simulink model "Smart_Grid_2"  (R2024b)
settings: Solver=FixedStepAuto  StartTime=0.0  StopTime=0.5  FixedStep=1e-5  RelTol=1e-3
undefined symbols (not defined in the file): Ion, Lithium
libraries: spsSeriesRLCBranchLib x76, spsRMSLib x65, spsIGBTDiodeLib x41, eeGeneralControl x36, slpidlib x34, spsThreePhaseVIMeasurementLib x32, spsVoltageMeasurementLib x18, simulink x16, spsCurrentMeasurementLib x15, spsThreePhaseBreakerLib x12, spsAlphaBetaZerotodq0Lib x12, spsPower3phPhasorLib x10
(part 2 of 8)

== system Smart_Grid_2/Residential Load 2 ==
  Demux5 : Demux  Outputs=3
  "Power (3ph, Phasor)" : spsPower3phPhasorLib/Power (3ph, Phasor)
      settings: LibrarySourceBlock=|
      | sps_lib/Sensors and Measurements/Power
      | (3ph, Phasor)
  RMS : spsRMSLib/RMS  TrueRMS=on  Freq=60  RMSInit=120  Ts=0
  RMS1 : spsRMSLib/RMS  TrueRMS=on  Freq=60  RMSInit=120  Ts=0
  Relay : Subsystem
  Residential Load 2 : spsThreePhaseParallelRLCLoadLib/Three-Phase Parallel RLC Load  LConnTagsString=A|B|C  Configuration=Y (grounded)  NominalVoltage=25e3  Vabc=[1e3 1e3 1e3]  Vabcp=[1e3 1e3 1e3]  NominalFrequency=50  UnbalancedPower=off  ActivePower=80e3  InductivePower=0  CapacitivePower=5000  Pabc=[10e3 9e3 11e3]  QLabc=[100 90 110]  QCabc=[100 90 110]  Pabcp=[10e3 9e3 11e3]  QLabcp=[100 90 110]  QCabcp=[100 90 110]  Measurements=None  LoadType=constant Z
  Scope : Scope  NumInputPorts=2
  Three-Phase V-I Measurement9 : spsThreePhaseVIMeasurementLib/Three-Phase V-I Measurement  VoltageMeasurement=phase-to-ground  SetLabelV=off  LabelV=Residential_2_Voltage  Vpu=off  VpuLL=off  CurrentMeasurement=yes  SetLabelI=off  LabelI=Residential_2_Current  Ipu=off  Pbase=100e6  Vbase=500e3  OutputType=Complex  PhasorSimulation=off  PSBequivalent=0
  Three-Phase Breaker : spsThreePhaseBreakerLib/Three-Phase Breaker  InitialState=closed  SwitchA=on  SwitchB=on  SwitchC=on  SwitchTimes="[1/60  5/60]"  External=on  BreakerResistance=0.001  SnubberResistance=1e8  SnubberCapacitance=inf  Measurements=Breaker voltages and currents
  Unit Delay2 : UnitDelay  SampleTime=0.001  HasFrameUpgradeWarning=on
  A : PMIOPort  Side=Left
  B : PMIOPort  Port=2  Side=Left
  C : PMIOPort  Port=3  Side=Left
  wires:
  Demux5/1 -> Relay/1(In1)
  Unit Delay2/1 -> Demux5/1
  Three-Phase V-I Measurement9/1 -> "Power (3ph, Phasor)"/1
  Three-Phase V-I Measurement9/2 -> "Power (3ph, Phasor)"/2, Unit Delay2/1
  Demux5/2 -> Relay/2(In2)
  Relay/1(Out1) -> Three-Phase Breaker/1
  "Power (3ph, Phasor)"/2 -> RMS1/1
  Demux5/3 -> Relay/3(In3)
  RMS1/1 -> Scope/2
  "Power (3ph, Phasor)"/1 -> RMS/1
  RMS/1 -> Scope/1
  connections:
  Three-Phase V-I Measurement9/LConn1 -- A/RConn1
  Three-Phase V-I Measurement9/LConn3 -- C/RConn1
  Three-Phase V-I Measurement9/LConn2 -- B/RConn1
  Three-Phase V-I Measurement9/RConn2 -- Three-Phase Breaker/LConn2
  Three-Phase Breaker/RConn2 -- Residential Load 2/LConn2
  Three-Phase Breaker/RConn1 -- Residential Load 2/LConn1
  Three-Phase V-I Measurement9/RConn3 -- Three-Phase Breaker/LConn3
  Three-Phase V-I Measurement9/RConn1 -- Three-Phase Breaker/LConn1
  Three-Phase Breaker/RConn3 -- Residential Load 2/LConn3

== system Smart_Grid_2/Residential Load 3 ==
  Demux5 : Demux  Outputs=3
  "Power (3ph, Phasor)" : spsPower3phPhasorLib/Power (3ph, Phasor)
      settings: LibrarySourceBlock=|
      | sps_lib/Sensors and Measurements/Power
      | (3ph, Phasor)
  RMS : spsRMSLib/RMS  TrueRMS=on  Freq=60  RMSInit=120  Ts=0
  RMS1 : spsRMSLib/RMS  TrueRMS=on  Freq=60  RMSInit=120  Ts=0
  Relay : Subsystem
  Residential Load 3 : spsThreePhaseParallelRLCLoadLib/Three-Phase Parallel RLC Load  LConnTagsString=A|B|C  Configuration=Y (grounded)  NominalVoltage=25e3  Vabc=[1e3 1e3 1e3]  Vabcp=[1e3 1e3 1e3]  NominalFrequency=50  UnbalancedPower=off  ActivePower=50e3  InductivePower=5000  CapacitivePower=0  Pabc=[10e3 9e3 11e3]  QLabc=[100 90 110]  QCabc=[100 90 110]  Pabcp=[10e3 9e3 11e3]  QLabcp=[100 90 110]  QCabcp=[100 90 110]  Measurements=None  LoadType=constant Z
  Scope : Scope  NumInputPorts=2
  Three-Phase V-I Measurement10 : spsThreePhaseVIMeasurementLib/Three-Phase V-I Measurement  VoltageMeasurement=phase-to-ground  SetLabelV=off  LabelV=Residential_3_Voltage  Vpu=off  VpuLL=off  CurrentMeasurement=yes  SetLabelI=off  LabelI=Residential_3_Current  Ipu=off  Pbase=100e6  Vbase=500e3  OutputType=Complex  PhasorSimulation=off  PSBequivalent=0
  Three-Phase Breaker : spsThreePhaseBreakerLib/Three-Phase Breaker  InitialState=closed  SwitchA=on  SwitchB=on  SwitchC=on  SwitchTimes="[1/60  5/60]"  External=on  BreakerResistance=0.001  SnubberResistance=1e8  SnubberCapacitance=inf  Measurements=Breaker voltages and currents
  Unit Delay2 : UnitDelay  SampleTime=0.001  HasFrameUpgradeWarning=on
  A : PMIOPort  Side=Left
  B : PMIOPort  Port=2  Side=Left
  C : PMIOPort  Port=3  Side=Left
  wires:
  Demux5/1 -> Relay/1(In1)
  Unit Delay2/1 -> Demux5/1
  Three-Phase V-I Measurement10/1 -> "Power (3ph, Phasor)"/1
  Three-Phase V-I Measurement10/2 -> "Power (3ph, Phasor)"/2, Unit Delay2/1
  Demux5/2 -> Relay/2(In2)
  Relay/1(Out1) -> Three-Phase Breaker/1
  "Power (3ph, Phasor)"/2 -> RMS1/1
  Demux5/3 -> Relay/3(In3)
  RMS1/1 -> Scope/2
  "Power (3ph, Phasor)"/1 -> RMS/1
  RMS/1 -> Scope/1
  connections:
  Three-Phase V-I Measurement10/LConn3 -- C/RConn1
  Three-Phase V-I Measurement10/LConn2 -- B/RConn1
  Three-Phase V-I Measurement10/LConn1 -- A/RConn1
  Three-Phase Breaker/LConn2 -- Three-Phase V-I Measurement10/RConn2
  Three-Phase Breaker/RConn2 -- Residential Load 3/LConn2
  Three-Phase Breaker/RConn1 -- Residential Load 3/LConn1
  Three-Phase Breaker/LConn3 -- Three-Phase V-I Measurement10/RConn3
  Three-Phase Breaker/LConn1 -- Three-Phase V-I Measurement10/RConn1
  Three-Phase Breaker/RConn3 -- Residential Load 3/LConn3

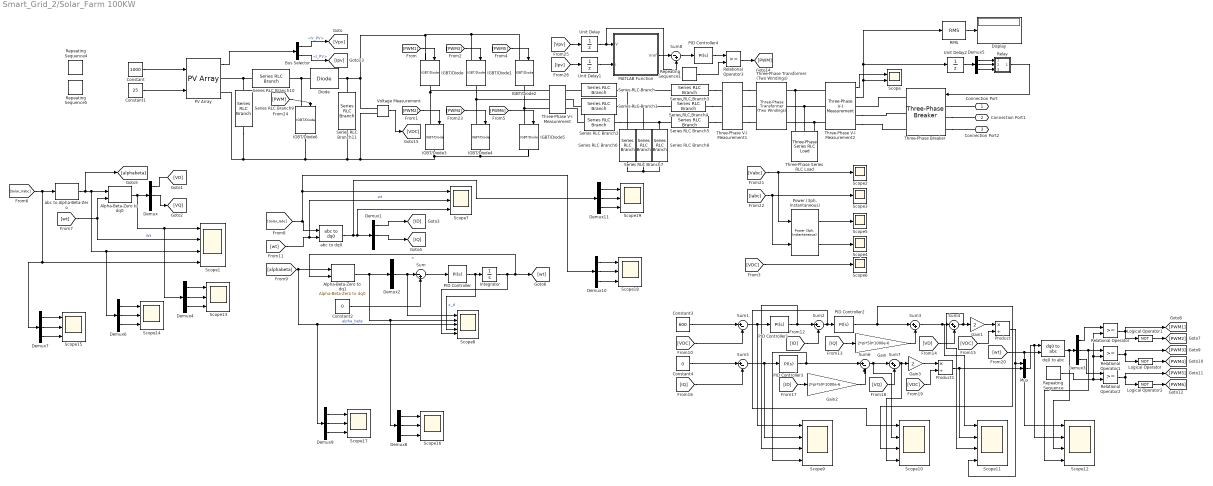
== system Smart_Grid_2/Solar_Farm 100KW ==
  Alpha-Beta-Zero to dq0 : spsAlphaBetaZerotodq0Lib/Alpha-Beta-Zero to dq0  Alignment=90 degrees behind phase A axis
  Alpha-Beta-Zero to dq1 : spsAlphaBetaZerotodq0Lib/Alpha-Beta-Zero to dq0  Alignment=90 degrees behind phase A axis
  Bus Selector : BusSelector  OutputSignals=V_PV,I_PV
  Constant : Constant  Value=1000
  Constant1 : Constant  Value=25
  Constant2 : Constant  Value=0
  Constant3 : Constant  Value=600
  Constant4 : Constant  Value=0
  Demux{,1..11} (12 alike) : Demux  Outputs=3
  Diode : spsDiodeLib/Diode  Ron=0.001  Lon=0  Vf=0.8  IC=0  UseSnubber=0  Rs=500  Cs=250e-9  Measurements=off
  Display : Display
  Gain : Gain  Gain=2*pi*50*1000e-6
  Gain1 : Gain  Gain=2
  Gain2 : Gain  Gain=2*pi*50*1000e-6
  Gain3 : Gain  Gain=2
  IGBT/Diode{,1..6} (7 alike) : spsIGBTDiodeLib/IGBT//Diode  Ron=1e-3  Rs=1e5  Cs=inf  Measurements=off
  Integrator : Integrator
  Logical Operator : Logic  Operator=NOT  AllPortsSameDT=off  OutDataTypeStr=boolean
  Logical Operator1 : Logic  Operator=NOT  AllPortsSameDT=off  OutDataTypeStr=boolean
  Logical Operator2 : Logic  Operator=NOT  AllPortsSameDT=off  OutDataTypeStr=boolean
  MATLAB Function : MATLAB Function  TreatAsAtomicUnit=on
  Mux : Mux  Inputs=3
  PID Controller : slpidlib/PID Controller  Controller=PI  Form=Parallel  TimeDomain=Continuous-time  UseExternalTs=off  SampleTime=-1  IntegratorMethod=Forward Euler  FilterMethod=Forward Euler  ControllerParametersSource=internal  P=10  I=50000  UseKiTs=off  D=0  UseExternalDerivativeSource=off  N=100  UseFilter=on  TunerSelectOption=Transfer Function Based (PID Tuner App)  InitialConditionSource=internal  InitialConditionForIntegrator=0  InitialConditionForFilter=0  DifferentiatorICPrevScaledInput=0  ExternalReset=none  TrackingMode=off  Kt=1  LimitOutput=off  SatLimitsSource=internal  UpperSaturationLimit=inf  LowerSaturationLimit=-inf  LinearizeAsGain=on  AntiWindupMode=none  Kb=1  LimitIntegrator=off  UpperIntegratorSaturationLimit=inf  LowerIntegratorSaturationLimit=-inf  POutMin=[]  POutMax=[]  IOutMin=[]  IOutMax=[]  DOutMin=[]  DOutMax=[]  NOutMin=[]  NOutMax=[]  SumOutMin=[]  SumOutMax=[]  SaturationOutMin=[]  SaturationOutMax=[]  PParamMin=[]  PParamMax=[]  IParamMin=[]  IParamMax=[]  DParamMin=[]  DParamMax=[]  NParamMin=[]  NParamMax=[]  KbParamMin=[]  KbParamMax=[]  KtParamMin=[]  KtParamMax=[]  KbOutMin=[]  KbOutMax=[]  KtOutMin=[]  KtOutMax=[]  IntegratorOutMin=[]  IntegratorOutMax=[]  FilterOutMin=[]  FilterOutMax=[]  SumI1OutMin=[]  SumI1OutMax=[]  SumI2OutMin=[]  SumI2OutMax=[]  SumI3OutMin=[]  SumI3OutMax=[]  SumI4OutMin=[]  SumI4OutMax=[]  SumDOutMin=[]  SumDOutMax=[]  DifferentiatorOutMin=[]  DifferentiatorOutMax=[]  FilterDiffOutCoefMin=[]  FilterDiffOutCoefMax=[]  ReciprocalOutMin=[]  ReciprocalOutMax=[]  SumDenOutMin=[]  SumDenOutMax=[]  SumNumOutMin=[]  SumNumOutMax=[]  DivideOutMin=[]  DivideOutMax=[]  UdiffTsProdOutMin=[]  UdiffTsProdOutMax=[]  NTsProdOutMin=[]  NTsProdOutMax=[]  UintegralTsProdOutMin=[]  UintegralTsProdOutMax=[]  UngainTsProdOutMin=[]  UngainTsProdOutMax=[]  ClampingZeroOutDataTypeStr=Inherit: Inherit via back propagation  ClampingZeroOutMin=[]  ClampingZeroOutMax=[]  FilterDenConstantOutDataTypeStr=Inherit: Inherit via back propagation  FilterDenConstantOutMin=[]  FilterDenConstantOutMax=[]  PCopyOutDataTypeStr=Inherit: Inherit via back propagation  PCopyOutMin=[]  PCopyOutMax=[]  NCopyOutDataTypeStr=Inherit: Inherit via back propagation  NCopyOutMin=[]  NCopyOutMax=[]  IntegratorContinuousStateAttributes=''  IntegratorStateMustResolveToSignalObject=off  IntegratorRTWStateStorageClass=Auto  FilterContinuousStateAttributes=''  FilterStateMustResolveToSignalObject=off  FilterRTWStateStorageClass=Auto  ParallelPVariant=InternalParameters  IdealPVariant=Disabled  IVariant=InternalParameters  DVariant=Disabled  IntegratorVariant=Continuous  SatVariant=Disabled  AWVariant=Passthrough  PCopyVariant=Disabled  TRVariant=Disabled  FdbkBlocksVariant=Forward  IdealPFdbkVariant=Disabled  SatFdbkVariant=Disabled  DerivativeFilterVariant=Disabled  NVariant=Disabled  NCopyVariant=Disabled_SignalSpec  FilterICVariant=Disabled  IntegratorICVariant=InternalICs  ExternalResetVariant=Disabled  TRSumVariant=Passthrough  SumFdbkVariant=Disabled  SumVariant=Sum_PI  TsampFilterVariant=InternalTs  TsampNgainVariant=Passthrough  TsampIntegralVariant=Disabled_SignalSpec  ExternalSaturationOutDataTypeStr=Inherit: Same as second input  DerivativeSourceVariant=Disabled  PreIntVariant=InternalPreInt
  PID Controller1 : slpidlib/PID Controller  Controller=PI  Form=Parallel  TimeDomain=Continuous-time  UseExternalTs=off  SampleTime=-1  IntegratorMethod=Forward Euler  FilterMethod=Forward Euler  ControllerParametersSource=internal  P=0.25  I=300  UseKiTs=off  D=0  UseExternalDerivativeSource=off  N=100  UseFilter=on  TunerSelectOption=Transfer Function Based (PID Tuner App)  InitialConditionSource=internal  InitialConditionForIntegrator=0  InitialConditionForFilter=0  DifferentiatorICPrevScaledInput=0  ExternalReset=none  TrackingMode=off  Kt=1  LimitOutput=off  SatLimitsSource=internal  UpperSaturationLimit=inf  LowerSaturationLimit=-inf  LinearizeAsGain=on  AntiWindupMode=none  Kb=1  LimitIntegrator=off  UpperIntegratorSaturationLimit=inf  LowerIntegratorSaturationLimit=-inf  POutMin=[]  POutMax=[]  IOutMin=[]  IOutMax=[]  DOutMin=[]  DOutMax=[]  NOutMin=[]  NOutMax=[]  SumOutMin=[]  SumOutMax=[]  SaturationOutMin=[]  SaturationOutMax=[]  PParamMin=[]  PParamMax=[]  IParamMin=[]  IParamMax=[]  DParamMin=[]  DParamMax=[]  NParamMin=[]  NParamMax=[]  KbParamMin=[]  KbParamMax=[]  KtParamMin=[]  KtParamMax=[]  KbOutMin=[]  KbOutMax=[]  KtOutMin=[]  KtOutMax=[]  IntegratorOutMin=[]  IntegratorOutMax=[]  FilterOutMin=[]  FilterOutMax=[]  SumI1OutMin=[]  SumI1OutMax=[]  SumI2OutMin=[]  SumI2OutMax=[]  SumI3OutMin=[]  SumI3OutMax=[]  SumI4OutMin=[]  SumI4OutMax=[]  SumDOutMin=[]  SumDOutMax=[]  DifferentiatorOutMin=[]  DifferentiatorOutMax=[]  FilterDiffOutCoefMin=[]  FilterDiffOutCoefMax=[]  ReciprocalOutMin=[]  ReciprocalOutMax=[]  SumDenOutMin=[]  SumDenOutMax=[]  SumNumOutMin=[]  SumNumOutMax=[]  DivideOutMin=[]  DivideOutMax=[]  UdiffTsProdOutMin=[]  UdiffTsProdOutMax=[]  NTsProdOutMin=[]  NTsProdOutMax=[]  UintegralTsProdOutMin=[]  UintegralTsProdOutMax=[]  UngainTsProdOutMin=[]  UngainTsProdOutMax=[]  ClampingZeroOutDataTypeStr=Inherit: Inherit via back propagation  ClampingZeroOutMin=[]  ClampingZeroOutMax=[]  FilterDenConstantOutDataTypeStr=Inherit: Inherit via back propagation  FilterDenConstantOutMin=[]  FilterDenConstantOutMax=[]  PCopyOutDataTypeStr=Inherit: Inherit via back propagation  PCopyOutMin=[]  PCopyOutMax=[]  NCopyOutDataTypeStr=Inherit: Inherit via back propagation  NCopyOutMin=[]  NCopyOutMax=[]  IntegratorContinuousStateAttributes=''  IntegratorStateMustResolveToSignalObject=off  IntegratorRTWStateStorageClass=Auto  FilterContinuousStateAttributes=''  FilterStateMustResolveToSignalObject=off  FilterRTWStateStorageClass=Auto  ParallelPVariant=InternalParameters  IdealPVariant=Disabled  IVariant=InternalParameters  DVariant=Disabled  IntegratorVariant=Continuous  SatVariant=Disabled  AWVariant=Passthrough  PCopyVariant=Disabled  TRVariant=Disabled  FdbkBlocksVariant=Forward  IdealPFdbkVariant=Disabled  SatFdbkVariant=Disabled  DerivativeFilterVariant=Disabled  NVariant=Disabled  NCopyVariant=Disabled_SignalSpec  FilterICVariant=Disabled  IntegratorICVariant=InternalICs  ExternalResetVariant=Disabled  TRSumVariant=Passthrough  SumFdbkVariant=Disabled  SumVariant=Sum_PI  TsampFilterVariant=InternalTs  TsampNgainVariant=Passthrough  TsampIntegralVariant=Disabled_SignalSpec  ExternalSaturationOutDataTypeStr=Inherit: Same as second input  DerivativeSourceVariant=Disabled  PreIntVariant=InternalPreInt
  PID Controller2 : slpidlib/PID Controller  Controller=PI  Form=Parallel  TimeDomain=Continuous-time  UseExternalTs=off  SampleTime=-1  IntegratorMethod=Forward Euler  FilterMethod=Forward Euler  ControllerParametersSource=internal  P=10  I=20  UseKiTs=off  D=0  UseExternalDerivativeSource=off  N=100  UseFilter=on  TunerSelectOption=Transfer Function Based (PID Tuner App)  InitialConditionSource=internal  InitialConditionForIntegrator=0  InitialConditionForFilter=0  DifferentiatorICPrevScaledInput=0  ExternalReset=none  TrackingMode=off  Kt=1  LimitOutput=off  SatLimitsSource=internal  UpperSaturationLimit=inf  LowerSaturationLimit=-inf  LinearizeAsGain=on  AntiWindupMode=none  Kb=1  LimitIntegrator=off  UpperIntegratorSaturationLimit=inf  LowerIntegratorSaturationLimit=-inf  POutMin=[]  POutMax=[]  IOutMin=[]  IOutMax=[]  DOutMin=[]  DOutMax=[]  NOutMin=[]  NOutMax=[]  SumOutMin=[]  SumOutMax=[]  SaturationOutMin=[]  SaturationOutMax=[]  PParamMin=[]  PParamMax=[]  IParamMin=[]  IParamMax=[]  DParamMin=[]  DParamMax=[]  NParamMin=[]  NParamMax=[]  KbParamMin=[]  KbParamMax=[]  KtParamMin=[]  KtParamMax=[]  KbOutMin=[]  KbOutMax=[]  KtOutMin=[]  KtOutMax=[]  IntegratorOutMin=[]  IntegratorOutMax=[]  FilterOutMin=[]  FilterOutMax=[]  SumI1OutMin=[]  SumI1OutMax=[]  SumI2OutMin=[]  SumI2OutMax=[]  SumI3OutMin=[]  SumI3OutMax=[]  SumI4OutMin=[]  SumI4OutMax=[]  SumDOutMin=[]  SumDOutMax=[]  DifferentiatorOutMin=[]  DifferentiatorOutMax=[]  FilterDiffOutCoefMin=[]  FilterDiffOutCoefMax=[]  ReciprocalOutMin=[]  ReciprocalOutMax=[]  SumDenOutMin=[]  SumDenOutMax=[]  SumNumOutMin=[]  SumNumOutMax=[]  DivideOutMin=[]  DivideOutMax=[]  UdiffTsProdOutMin=[]  UdiffTsProdOutMax=[]  NTsProdOutMin=[]  NTsProdOutMax=[]  UintegralTsProdOutMin=[]  UintegralTsProdOutMax=[]  UngainTsProdOutMin=[]  UngainTsProdOutMax=[]  ClampingZeroOutDataTypeStr=Inherit: Inherit via back propagation  ClampingZeroOutMin=[]  ClampingZeroOutMax=[]  FilterDenConstantOutDataTypeStr=Inherit: Inherit via back propagation  FilterDenConstantOutMin=[]  FilterDenConstantOutMax=[]  PCopyOutDataTypeStr=Inherit: Inherit via back propagation  PCopyOutMin=[]  PCopyOutMax=[]  NCopyOutDataTypeStr=Inherit: Inherit via back propagation  NCopyOutMin=[]  NCopyOutMax=[]  IntegratorContinuousStateAttributes=''  IntegratorStateMustResolveToSignalObject=off  IntegratorRTWStateStorageClass=Auto  FilterContinuousStateAttributes=''  FilterStateMustResolveToSignalObject=off  FilterRTWStateStorageClass=Auto  ParallelPVariant=InternalParameters  IdealPVariant=Disabled  IVariant=InternalParameters  DVariant=Disabled  IntegratorVariant=Continuous  SatVariant=Disabled  AWVariant=Passthrough  PCopyVariant=Disabled  TRVariant=Disabled  FdbkBlocksVariant=Forward  IdealPFdbkVariant=Disabled  SatFdbkVariant=Disabled  DerivativeFilterVariant=Disabled  NVariant=Disabled  NCopyVariant=Disabled_SignalSpec  FilterICVariant=Disabled  IntegratorICVariant=InternalICs  ExternalResetVariant=Disabled  TRSumVariant=Passthrough  SumFdbkVariant=Disabled  SumVariant=Sum_PI  TsampFilterVariant=InternalTs  TsampNgainVariant=Passthrough  TsampIntegralVariant=Disabled_SignalSpec  ExternalSaturationOutDataTypeStr=Inherit: Same as second input  DerivativeSourceVariant=Disabled  PreIntVariant=InternalPreInt
  PID Controller3 : slpidlib/PID Controller  Controller=PI  Form=Parallel  TimeDomain=Continuous-time  UseExternalTs=off  SampleTime=-1  IntegratorMethod=Forward Euler  FilterMethod=Forward Euler  ControllerParametersSource=internal  P=10  I=20  UseKiTs=off  D=0  UseExternalDerivativeSource=off  N=100  UseFilter=on  TunerSelectOption=Transfer Function Based (PID Tuner App)  InitialConditionSource=internal  InitialConditionForIntegrator=0  InitialConditionForFilter=0  DifferentiatorICPrevScaledInput=0  ExternalReset=none  TrackingMode=off  Kt=1  LimitOutput=off  SatLimitsSource=internal  UpperSaturationLimit=inf  LowerSaturationLimit=-inf  LinearizeAsGain=on  AntiWindupMode=none  Kb=1  LimitIntegrator=off  UpperIntegratorSaturationLimit=inf  LowerIntegratorSaturationLimit=-inf  POutMin=[]  POutMax=[]  IOutMin=[]  IOutMax=[]  DOutMin=[]  DOutMax=[]  NOutMin=[]  NOutMax=[]  SumOutMin=[]  SumOutMax=[]  SaturationOutMin=[]  SaturationOutMax=[]  PParamMin=[]  PParamMax=[]  IParamMin=[]  IParamMax=[]  DParamMin=[]  DParamMax=[]  NParamMin=[]  NParamMax=[]  KbParamMin=[]  KbParamMax=[]  KtParamMin=[]  KtParamMax=[]  KbOutMin=[]  KbOutMax=[]  KtOutMin=[]  KtOutMax=[]  IntegratorOutMin=[]  IntegratorOutMax=[]  FilterOutMin=[]  FilterOutMax=[]  SumI1OutMin=[]  SumI1OutMax=[]  SumI2OutMin=[]  SumI2OutMax=[]  SumI3OutMin=[]  SumI3OutMax=[]  SumI4OutMin=[]  SumI4OutMax=[]  SumDOutMin=[]  SumDOutMax=[]  DifferentiatorOutMin=[]  DifferentiatorOutMax=[]  FilterDiffOutCoefMin=[]  FilterDiffOutCoefMax=[]  ReciprocalOutMin=[]  ReciprocalOutMax=[]  SumDenOutMin=[]  SumDenOutMax=[]  SumNumOutMin=[]  SumNumOutMax=[]  DivideOutMin=[]  DivideOutMax=[]  UdiffTsProdOutMin=[]  UdiffTsProdOutMax=[]  NTsProdOutMin=[]  NTsProdOutMax=[]  UintegralTsProdOutMin=[]  UintegralTsProdOutMax=[]  UngainTsProdOutMin=[]  UngainTsProdOutMax=[]  ClampingZeroOutDataTypeStr=Inherit: Inherit via back propagation  ClampingZeroOutMin=[]  ClampingZeroOutMax=[]  FilterDenConstantOutDataTypeStr=Inherit: Inherit via back propagation  FilterDenConstantOutMin=[]  FilterDenConstantOutMax=[]  PCopyOutDataTypeStr=Inherit: Inherit via back propagation  PCopyOutMin=[]  PCopyOutMax=[]  NCopyOutDataTypeStr=Inherit: Inherit via back propagation  NCopyOutMin=[]  NCopyOutMax=[]  IntegratorContinuousStateAttributes=''  IntegratorStateMustResolveToSignalObject=off  IntegratorRTWStateStorageClass=Auto  FilterContinuousStateAttributes=''  FilterStateMustResolveToSignalObject=off  FilterRTWStateStorageClass=Auto  ParallelPVariant=InternalParameters  IdealPVariant=Disabled  IVariant=InternalParameters  DVariant=Disabled  IntegratorVariant=Continuous  SatVariant=Disabled  AWVariant=Passthrough  PCopyVariant=Disabled  TRVariant=Disabled  FdbkBlocksVariant=Forward  IdealPFdbkVariant=Disabled  SatFdbkVariant=Disabled  DerivativeFilterVariant=Disabled  NVariant=Disabled  NCopyVariant=Disabled_SignalSpec  FilterICVariant=Disabled  IntegratorICVariant=InternalICs  ExternalResetVariant=Disabled  TRSumVariant=Passthrough  SumFdbkVariant=Disabled  SumVariant=Sum_PI  TsampFilterVariant=InternalTs  TsampNgainVariant=Passthrough  TsampIntegralVariant=Disabled_SignalSpec  ExternalSaturationOutDataTypeStr=Inherit: Same as second input  DerivativeSourceVariant=Disabled  PreIntVariant=InternalPreInt
  PID Controller4 : slpidlib/PID Controller  Controller=PI  Form=Parallel  TimeDomain=Continuous-time  UseExternalTs=off  SampleTime=-1  IntegratorMethod=Forward Euler  FilterMethod=Forward Euler  ControllerParametersSource=internal  P=0.005  I=0.001  UseKiTs=off  D=0  UseExternalDerivativeSource=off  N=100  UseFilter=on  TunerSelectOption=Transfer Function Based (PID Tuner App)  InitialConditionSource=internal  InitialConditionForIntegrator=0  InitialConditionForFilter=0  DifferentiatorICPrevScaledInput=0  ExternalReset=none  TrackingMode=off  Kt=1  LimitOutput=on  SatLimitsSource=internal  UpperSaturationLimit=0.95  LowerSaturationLimit=0  LinearizeAsGain=on  AntiWindupMode=none  Kb=1  LimitIntegrator=off  UpperIntegratorSaturationLimit=inf  LowerIntegratorSaturationLimit=-inf  POutMin=[]  POutMax=[]  IOutMin=[]  IOutMax=[]  DOutMin=[]  DOutMax=[]  NOutMin=[]  NOutMax=[]  SumOutMin=[]  SumOutMax=[]  SaturationOutMin=[]  SaturationOutMax=[]  PParamMin=[]  PParamMax=[]  IParamMin=[]  IParamMax=[]  DParamMin=[]  DParamMax=[]  NParamMin=[]  NParamMax=[]  KbParamMin=[]  KbParamMax=[]  KtParamMin=[]  KtParamMax=[]  KbOutMin=[]  KbOutMax=[]  KtOutMin=[]  KtOutMax=[]  IntegratorOutMin=[]  IntegratorOutMax=[]  FilterOutMin=[]  FilterOutMax=[]  SumI1OutMin=[]  SumI1OutMax=[]  SumI2OutMin=[]  SumI2OutMax=[]  SumI3OutMin=[]  SumI3OutMax=[]  SumI4OutMin=[]  SumI4OutMax=[]  SumDOutMin=[]  SumDOutMax=[]  DifferentiatorOutMin=[]  DifferentiatorOutMax=[]  FilterDiffOutCoefMin=[]  FilterDiffOutCoefMax=[]  ReciprocalOutMin=[]  ReciprocalOutMax=[]  SumDenOutMin=[]  SumDenOutMax=[]  SumNumOutMin=[]  SumNumOutMax=[]  DivideOutMin=[]  DivideOutMax=[]  UdiffTsProdOutMin=[]  UdiffTsProdOutMax=[]  NTsProdOutMin=[]  NTsProdOutMax=[]  UintegralTsProdOutMin=[]  UintegralTsProdOutMax=[]  UngainTsProdOutMin=[]  UngainTsProdOutMax=[]  ClampingZeroOutDataTypeStr=Inherit: Inherit via back propagation  ClampingZeroOutMin=[]  ClampingZeroOutMax=[]  FilterDenConstantOutDataTypeStr=Inherit: Inherit via back propagation  FilterDenConstantOutMin=[]  FilterDenConstantOutMax=[]  PCopyOutDataTypeStr=Inherit: Inherit via back propagation  PCopyOutMin=[]  PCopyOutMax=[]  NCopyOutDataTypeStr=Inherit: Inherit via back propagation  NCopyOutMin=[]  NCopyOutMax=[]  IntegratorContinuousStateAttributes=''  IntegratorStateMustResolveToSignalObject=off  IntegratorRTWStateStorageClass=Auto  FilterContinuousStateAttributes=''  FilterStateMustResolveToSignalObject=off  FilterRTWStateStorageClass=Auto  ParallelPVariant=InternalParameters  IdealPVariant=Disabled  IVariant=InternalParameters  DVariant=Disabled  IntegratorVariant=Continuous  SatVariant=Enabled  AWVariant=Passthrough  PCopyVariant=Disabled  TRVariant=Disabled  FdbkBlocksVariant=Forward  IdealPFdbkVariant=Disabled  SatFdbkVariant=Disabled  DerivativeFilterVariant=Disabled  NVariant=Disabled  NCopyVariant=Disabled_SignalSpec  FilterICVariant=Disabled  IntegratorICVariant=InternalICs  ExternalResetVariant=Disabled  TRSumVariant=Passthrough  SumFdbkVariant=Disabled  SumVariant=Sum_PI  TsampFilterVariant=InternalTs  TsampNgainVariant=Passthrough  TsampIntegralVariant=Disabled_SignalSpec  ExternalSaturationOutDataTypeStr=Inherit: Same as second input  DerivativeSourceVariant=Disabled  PreIntVariant=InternalPreInt
  PV Array : spsPVArrayLib/PV Array  Npar=47  Nser=10  PlotType=array @ 25 deg.C & specified irradiances  S_vec="[ 1000  500  100 ]"  Temp_C_vec="[ 45 25  ]"  ModuleName=Solartech Renewables STR215  PlotWhenSelected=off  Pm=214.963  Ncell=60  Voc=36  Isc=7.73  Vm=28.7  Im=7.49  beta_Voc_pc=-0.41  alpha_Isc_pc=0.05  beta_Voc=-0.1476  alpha_Isc=0.003865  IL=7.8848  I0=1.3153e-09  nI=1.0373  Rsh=5284.6435  Rs=0.36886  RobustModel=off  RobustCellTemperature=313.3991  BAL=on  Tc=1e-6  Tfilter=5e-5
  "Power (3ph, Instantaneous)" : spsPower3phInstantaneousLib/Power (3ph, Instantaneous)
  Product : Product  Inputs=*/
  Product1 : Product  Inputs=*/
  RMS : spsRMSLib/RMS  TrueRMS=on  Freq=50  RMSInit=0  Ts=0.001
  Relational Operator{,1..3} (4 alike) : RelationalOperator  OutDataTypeStr=boolean  RndMeth=Simplest  InputSameDT=off
  Relay : Subsystem
  Repeating Sequence : simulink/Sources/Repeating Sequence  rep_seq_t=[0 0.00005 0.0001]  rep_seq_y=[-1 1 -1]
  Repeating Sequence1 : simulink/Sources/Repeating Sequence  rep_seq_t=[0 0.0002]  rep_seq_y=[0 1]
  Repeating Sequence4 : simulink/Sources/Repeating Sequence  rep_seq_t=|  rep_seq_y=|
      rep_seq_t=|
      | [0
      | 0.050505051
      | 0.101010101
      | 0.151515152
      | 0.202020202
      | 0.252525253
      | 0.303030303
      | 0.353535354
      | 0.404040404
      | 0.454545455
      | 0.505050505
      | 0.555555556
      | 0.606060606
      | 0.656565657
      | 0.707070707
      | 0.757575758
      | 0.808080808
      | 0.858585859
      | 0.909090909
      | 0.95959596
      | 1.01010101
      | 1.060606061
      | 1.111111111
      | 1.161616162
      | 1.212121212
      | 1.262626263
      | 1.313131313
      | 1.363636364
      | 1.414141414
      | 1.464646465
      | 1.515151515
      | 1.565656566
      | 1.616161616
      | 1.666666667
      | 1.717171717
      | 1.767676768
      | 1.818181818
      | 1.868686869
      | 1.919191919
      | 1.96969697
      | 2.02020202
      | 2.070707071
      | 2.121212121
      | 2.171717172
      | 2.222222222
      | 2.272727273
      | 2.323232323
      | 2.373737374
      | 2.424242424
      | 2.474747475
      | 2.525252525
      | 2.575757576
      | 2.626262626
      | 2.676767677
      | 2.727272727
      | 2.777777778
      | 2.828282828
      | 2.878787879
      | 2.929292929
      | 2.97979798
      | 3.03030303
      | 3.080808081
      | 3.131313131
      | 3.181818182
      | 3.232323232
      | 3.282828283
      | 3.333333333
      | 3.383838384
      | 3.434343434
      | 3.484848485
      | 3.535353535
      | 3.585858586
      | 3.636363636
      | 3.686868687
      | 3.737373737
      | 3.787878788
      | 3.838383838
      | 3.888888889
      | 3.939393939
      | 3.98989899
      | 4.04040404
      | 4.090909091
      | 4.141414141
      | 4.191919192
      | 4.242424242
      | 4.292929293
      | 4.343434343
      | 4.393939394
      | 4.444444444
      | 4.494949495
      | 4.545454545
      | 4.595959596
      | 4.646464646
      | 4.696969697
      | 4.747474747
      | 4.797979798
      | 4.848484848
      | 4.898989899
      | 4.949494949
      | 5
      | ]
      rep_seq_y=|
      | [961.731225
      | 1045.11045
      | 1008.510311
      | 931.1104746
      | 1078.747978
      | 1059.848715
      | 904.7074666
      | 958.4820041
      | 947.434516
      | 1200.30114
      | 1066.976539
      | 1076.06026
      | 1093.154951
      | 1055.443451
      | 901.2390038
      | 1091.945745
      | 953.8403505
      | 0
      | 0
      | 0
      | 0
      | 0
      | 0
      | 0
      | 1000.207161
      | 1038.593515
      | 941.0686417
      | 500.4919759
      | 550.6758168
      | 939.0750316
      | 936.755036
      | 1086.548091
      | 1027.661514
      | 1076.95396
      | 1093.908545
      | 969.8802795
      | 900.0079837
      | 1039.498473
      | 350.3719924
      | 400.3916341
      | 420.2982665
      | 1029.138637
      | 960.2858986
      | 949.2673312
      | 1067.379392
      | 1058.456925
      | 986.3566657
      | 948.4318496
      | 942.3822613
      | 916.4479292
      | 1002.255686
      | 1068.546297
      | 1080.245726
      | 927.5500873
      | 967.3817546
      | 946.7661715
      | 998.0233465
      | 1036.639395
      | 1075.77624
      | 1099.604998
      | 910.8779584
      | 1053.351328
      | 1079.393791
      | 1002.654666
      | 1028.287667
      | 951.1786685
      | 974.5537092
      | 1024.300777
      | 998.6087208
      | 903.7161662
      | 1081.108921
      | 922.113608
      | 923.529757
      | 941.6210422
      | 984.1534846
      | 1046.704566
      | 1087.490012
      | 917.4050569
      | 1068.395551
      | 984.3349603
      | 1054.093286
      | 999.8107273
      | 917.4038553
      | 932.1890541
      | 951.4940944
      | 903.1694839
      | 964.5157871
      | 917.1253389
      | 954.3180431
      | 1071.497523
      | 935.2374128
      | 1056.905007
      | 1039.774892
      | 1055.449509
      | 984.8677414
      | 961.3374658
      | 1088.467992
      | 1058.226697
      | 970.9178907
      | 908.7847737
      | ]
  Repeating Sequence5 : simulink/Sources/Repeating Sequence  rep_seq_t=|  rep_seq_y=|
      rep_seq_t=|
      | [0
      | 0.050505051
      | 0.101010101
      | 0.151515152
      | 0.202020202
      | 0.252525253
      | 0.303030303
      | 0.353535354
      | 0.404040404
      | 0.454545455
      | 0.505050505
      | 0.555555556
      | 0.606060606
      | 0.656565657
      | 0.707070707
      | 0.757575758
      | 0.808080808
      | 0.858585859
      | 0.909090909
      | 0.95959596
      | 1.01010101
      | 1.060606061
      | 1.111111111
      | 1.161616162
      | 1.212121212
      | 1.262626263
      | 1.313131313
      | 1.363636364
      | 1.414141414
      | 1.464646465
      | 1.515151515
      | 1.565656566
      | 1.616161616
      | 1.666666667
      | 1.717171717
      | 1.767676768
      | 1.818181818
      | 1.868686869
      | 1.919191919
      | 1.96969697
      | 2.02020202
      | 2.070707071
      | 2.121212121
      | 2.171717172
      | 2.222222222
      | 2.272727273
      | 2.323232323
      | 2.373737374
      | 2.424242424
      | 2.474747475
      | 2.525252525
      | 2.575757576
      | 2.626262626
      | 2.676767677
      | 2.727272727
      | 2.777777778
      | 2.828282828
      | 2.878787879
      | 2.929292929
      | 2.97979798
      | 3.03030303
      | 3.080808081
      | 3.131313131
      | 3.181818182
      | 3.232323232
      | 3.282828283
      | 3.333333333
      | 3.383838384
      | 3.434343434
      | 3.484848485
      | 3.535353535
      | 3.585858586
      | 3.636363636
      | 3.686868687
      | 3.737373737
      | 3.787878788
      | 3.838383838
      | 3.888888889
      | 3.939393939
      | 3.98989899
      | 4.04040404
      | 4.090909091
      | 4.141414141
      | 4.191919192
      | 4.242424242
      | 4.292929293
      | 4.343434343
      | 4.393939394
      | 4.444444444
      | 4.494949495
      | 4.545454545
      | 4.595959596
      | 4.646464646
      | 4.696969697
      | 4.747474747
      | 4.797979798
      | 4.848484848
      | 4.898989899
      | 4.949494949
      | 5
      | ]
      rep_seq_y=|
      | [39.09040776
      | 33.78587594
      | 22.64735033
      | 39.07287359
      | 39.6979768
      | 38.77147184
      | 20.1126813
      | 32.72378376
      | 39.96246483
      | 35.82177272
      | 20.49274147
      | 30.62419618
      | 26.17597826
      | 38.66721226
      | 21.62717688
      | 21.97818325
      | 38.49825769
      | 36.17310767
      | 26.07943066
      | 28.57378964
      | 21.24308492
      | 26.36590257
      | 30.33391133
      | 29.99686413
      | 23.22998026
      | 38.53716796
      | 34.59986631
      | 24.14165098
      | 22.46973707
      | 25.64228662
      | 26.2700476
      | 38.78343151
      | 22.35947723
      | 26.17383265
      | 34.52437963
      | 27.85768308
      | 24.96183533
      | 24.06305535
      | 34.13520509
      | 29.27960727
      | 34.02958238
      | 31.19691976
      | 29.65246289
      | 22.82071168
      | 26.36562902
      | 37.00153111
      | 35.65458064
      | 23.04842989
      | 21.32587473
      | 30.35583122
      | 25.41212742
      | 32.94902261
      | 31.40546329
      | 27.39813642
      | 25.32840072
      | 24.51675606
      | 24.01324349
      | 30.88693234
      | 29.85790683
      | 27.80551597
      | 23.11303618
      | 30.90103153
      | 38.1204096
      | 37.66129424
      | 32.54190455
      | 25.87105192
      | 30.81157353
      | 33.91804655
      | 31.05518166
      | 37.05481269
      | 24.91683857
      | 28.99411247
      | 30.36584588
      | 22.30935985
      | 25.91476526
      | 21.87306052
      | 36.26770138
      | 23.15482256
      | 32.66810495
      | 33.93954581
      | 32.63846158
      | 28.38171681
      | 23.17522821
      | 25.70852908
      | 32.50154208
      | 34.83572597
      | 33.50995143
      | 36.59220243
      | 39.49654504
      | 26.69276484
      | 30.47625268
      | 24.22660242
      | 28.84239867
      | 24.12405795
      | 22.94119138
      | 22.51756848
      | 29.72937034
      | 31.48890937
      | 25.32014349
      | 20.45980854
      | ]
  Scope : Scope  NumInputPorts=2
  Scope{1,9..12} (5 alike) : Scope  NumInputPorts=4
  Scope{7,13..19} (8 alike) : Scope  NumInputPorts=3
  Scope{2..6} (5 alike) : Scope
  Scope8 : Scope  NumInputPorts=5
  Series RLC Branch{,1..5} (6 alike) : spsSeriesRLCBranchLib/Series RLC Branch  LConnTagsString=__new0  RConnTagsString=__new0  BranchType=RL  Resistance=1e-3  Inductance=500e-6  SetiL0=off  InitialCurrent=0  Capacitance=1e-6  Setx0=off  InitialVoltage=0  Measurements=None
  Series RLC Branch10 : spsSeriesRLCBranchLib/Series RLC Branch  LConnTagsString=__new0  RConnTagsString=__new0  BranchType=L  Resistance=1e-3  Inductance=1.45e-3  SetiL0=off  InitialCurrent=0  Capacitance=1000e-6  Setx0=off  InitialVoltage=0  Measurements=None
  Series RLC Branch11 : spsSeriesRLCBranchLib/Series RLC Branch  LConnTagsString=__new0  RConnTagsString=__new0  BranchType=C  Resistance=1e-3  Inductance=3227e-3  SetiL0=off  InitialCurrent=0  Capacitance=3227e-6  Setx0=off  InitialVoltage=0  Measurements=None
  Series RLC Branch6 : spsSeriesRLCBranchLib/Series RLC Branch  LConnTagsString=__new0  RConnTagsString=__new0  BranchType=RC  Resistance=1e-3  Inductance=500e-6  SetiL0=off  InitialCurrent=0  Capacitance=100e-6  Setx0=off  InitialVoltage=0  Measurements=None
  Series RLC Branch7 : spsSeriesRLCBranchLib/Series RLC Branch  LConnTagsString=__new0  RConnTagsString=__new0  BranchType=RC  Resistance=1e-3  Inductance=500e-6  SetiL0=off  InitialCurrent=0  Capacitance=100e-6  Setx0=off  InitialVoltage=0  Measurements=None
  Series RLC Branch8 : spsSeriesRLCBranchLib/Series RLC Branch  LConnTagsString=__new0  RConnTagsString=__new0  BranchType=RC  Resistance=1e-3  Inductance=500e-6  SetiL0=off  InitialCurrent=0  Capacitance=100e-6  Setx0=off  InitialVoltage=0  Measurements=None
  Series RLC Branch9 : spsSeriesRLCBranchLib/Series RLC Branch  LConnTagsString=__new0  RConnTagsString=__new0  BranchType=RC  Resistance=1e-3  Inductance=1e-3  SetiL0=off  InitialCurrent=0  Capacitance=100e-6  Setx0=off  InitialVoltage=0  Measurements=None
  Sum : Sum  Inputs=|-+
  Sum{1..2,5..6} (4 alike) : Sum  Inputs=|+-
  Sum3 : Sum  Inputs=|++
  Sum4 : Sum  Inputs=|++
  Sum7 : Sum  Inputs=|++
  Sum8 : Sum  Inputs=|-+
  Three-Phase Series RLC Load : spsThreePhaseSeriesRLCLoadLib/Three-Phase Series RLC Load  LConnTagsString=A|B|C  Configuration=Y (grounded)  NominalVoltage=25e3  Vabc=[1e3 1e3 1e3]  Vabcp=[1e3 1e3 1e3]  NominalFrequency=50  UnbalancedPower=off  ActivePower=100  InductivePower=0  CapacitivePower=10000  Pabc=[10e3 9e3 11e3]  QLabc=[100 90 110]  QCabc=[100 90 110]  Pabcp=[10e3 9e3 11e3]  QLabcp=[100 90 110]  QCabcp=[100 90 110]  Measurements=None  LoadType=constant Z
  Three-Phase Transformer (Two Windings) : spsThreePhaseTransformerTwoWindingsLib/Three-Phase Transformer (Two Windings)  Winding1Connection=Yg  Winding2Connection=Yg  CoreType=Three single-phase transformers  SetSaturation=off  Hysteresis=off  DataFile='hysteresis'  SetInitialFlux=off  Measurements=None  UNITS=pu  NominalPower=[ 25e6 , 50 ]  Winding1=[ 400 , 0 , 0 ]  Winding2=[ 25e3 , 0 , 0 ]  Rm=500  Lm=500  L0=0.5  Saturation=[ 0,0 ; 0.0024,1.2 ; 1.0,1.52 ]  InitialFluxes=[ 0.8 , -0.8 , 0.7 ]  BreakLoop=off  DiscreteSolver=Trapezoidal iterative  DataType=off  TransfoNumber=1
  Three-Phase V-I Measurement : spsThreePhaseVIMeasurementLib/Three-Phase V-I Measurement  VoltageMeasurement=no  SetLabelV=off  LabelV=Vabc  Vpu=off  VpuLL=off  CurrentMeasurement=yes  SetLabelI=on  LabelI=Solar_Iabc  Ipu=off  Pbase=100e6  Vbase=500e3  OutputType=Complex  PhasorSimulation=off  PSBequivalent=0
  Three-Phase V-I Measurement1 : spsThreePhaseVIMeasurementLib/Three-Phase V-I Measurement  VoltageMeasurement=phase-to-ground  SetLabelV=on  LabelV=Solar_Vabc  Vpu=off  VpuLL=off  CurrentMeasurement=no  SetLabelI=off  LabelI=Iabc  Ipu=off  Pbase=100e6  Vbase=500e3  OutputType=Complex  PhasorSimulation=off  PSBequivalent=0
  Three-Phase V-I Measurement2 : spsThreePhaseVIMeasurementLib/Three-Phase V-I Measurement  VoltageMeasurement=phase-to-ground  SetLabelV=off  LabelV=Vabc  Vpu=off  VpuLL=off  CurrentMeasurement=yes  SetLabelI=off  LabelI=Iabc  Ipu=off  Pbase=100e6  Vbase=500e3  OutputType=Complex  PhasorSimulation=off  PSBequivalent=0
  Three-Phase Breaker : spsThreePhaseBreakerLib/Three-Phase Breaker  InitialState=closed  SwitchA=on  SwitchB=on  SwitchC=on  SwitchTimes="[1/60  5/60]"  External=on  BreakerResistance=0.001  SnubberResistance=1e8  SnubberCapacitance=inf  Measurements=Breaker voltages and currents
  Unit Delay : UnitDelay  SampleTime=1e-4  HasFrameUpgradeWarning=on
  Unit Delay1 : UnitDelay  SampleTime=1e-4  HasFrameUpgradeWarning=on
  Unit Delay2 : UnitDelay  SampleTime=0.001  HasFrameUpgradeWarning=on
  Voltage Measurement : spsVoltageMeasurementLib/Voltage Measurement  PhasorSimulation=off  OutputType=Complex  PSBequivalent=0
  abc to Alpha-Beta-Zero : spsabctoAlphaBetaZeroLib/abc to Alpha-Beta-Zero
  abc to dq0 : spsabctodq0Lib/abc to dq0  Alignment=90 degrees behind phase A axis
  dq0 to abc : spsdq0toabcLib/dq0 to abc  Alignment=90 degrees behind phase A axis
  Connection Port : PMIOPort  Side=Right
  Connection Port1 : PMIOPort  Port=2  Side=Right
  Connection Port2 : PMIOPort  Port=3  Side=Right
  wires:
  Three-Phase V-I Measurement2/1 -> Scope/1
  [VDC] -> Scope6/1
  [Vabc] -> Scope2/1, "Power (3ph, Instantaneous)"/1
  "Power (3ph, Instantaneous)"/1 -> Scope5/1
  "Power (3ph, Instantaneous)"/2 -> Scope4/1
  [Iabc] -> Scope3/1, "Power (3ph, Instantaneous)"/2
  Demux3/3 -> Relational Operator2/1
  Repeating Sequence/1 -> Relational Operator/2, Relational Operator1/2, Relational Operator2/2
  Demux3/1 -> Relational Operator/1
  Demux3/2 -> Scope12/4, Relational Operator1/1
  dq0 to abc/1 -> Scope12/3, Demux3/1
  [ID] -> Gain2/1
  [VDC] -> Product1/2
  Sum5/1 -> Scope9/2, PID Controller3/1
  Constant4/1 -> Sum5/1
  [IQ] -> Sum5/2
  Sum6/1 -> Scope10/2, Sum7/1
  Sum7/1 -> Scope10/4, Gain3/1
  PID Controller3/1 -> Scope9/4, Sum6/1
  [VQ] -> Sum7/2
  Gain2/1 -> Sum6/2
  Gain3/1 -> Product1/1
  Demux2/2 -> Scope8/1, Sum/1
  [alphabeta] -> Demux9/1, Scope8/3, Alpha-Beta-Zero to dq1/1  "alpha_beta"
  Integrator/1 -> Scope8/5, Alpha-Beta-Zero to dq1/2, [wt]  "x"
  Constant2/1 -> Sum/2
  Sum/1 -> PID Controller/1
  PID Controller/1 -> Scope8/4, Integrator/1  "x_d"
  Demux1/2 -> [IQ]
  [Solar_Iabc] -> Demux10/1, Scope7/1, abc to dq0/1
  [wt] -> Scope7/2, abc to dq0/2  "wt"
  Demux1/1 -> [ID]
  PID Controller1/1 -> Scope9/3, Sum2/1
  Sum2/1 -> Scope10/1, PID Controller2/1
  [VDC] -> Sum1/2
  [VD] -> Sum4/2
  PID Controller2/1 -> Scope10/3, Sum3/1
  Sum3/1 -> Scope11/1, Sum4/1
  [IQ] -> Gain/1
  [VDC] -> Product/2
  Constant3/1 -> Sum1/1
  Gain/1 -> Sum3/2
  [ID] -> Sum2/2
  Gain1/1 -> Product/1
  Sum4/1 -> Scope11/3, Gain1/1
  Sum1/1 -> Scope9/1, PID Controller1/1
  Demux/1 -> [VD]
  Alpha-Beta-Zero to dq0/1 -> Demux/1, Demux4/1, Scope1/1
  [wt] -> Scope1/2, Alpha-Beta-Zero to dq0/2  "Wt"
  Demux/2 -> [VQ]
  Product1/1 -> Scope11/2, Mux/2
  Product/1 -> Scope11/4, Mux/1
  Mux/1 -> Scope12/2, dq0 to abc/1
  [wt] -> Scope12/1, dq0 to abc/2
  Logical Operator1/1 -> [PWM2]
  Logical Operator2/1 -> [PWM6]
  Relational Operator2/1 -> Logical Operator2/1, [PWM5]
  Relational Operator/1 -> Logical Operator1/1, [PWM1]
  Logical Operator/1 -> [PWM4]
  Relational Operator1/1 -> [PWM3], Logical Operator/1
  [PWM1] -> IGBT/Diode/1
  [PWM5] -> IGBT/Diode2/1
  [PWM4] -> IGBT/Diode4/1
  [PWM3] -> IGBT/Diode1/1
  [PWM6] -> IGBT/Diode5/1
  [PWM2] -> IGBT/Diode3/1
  Voltage Measurement/1 -> [VDC]
  Relational Operator3/1 -> [PWM]
  Sum8/1 -> PID Controller4/1
  [Ipv] -> Unit Delay1/1
  Repeating Sequence1/1 -> Relational Operator3/2
  Unit Delay/1 -> Sum8/2, MATLAB Function/1(V)
  [PWM] -> IGBT/Diode6/1
  PID Controller4/1 -> Relational Operator3/1
  PV Array/1 -> Bus Selector/1
  [Vpv] -> Unit Delay/1
  Bus Selector/1 -> [Vpv]  "<V_PV>"
  Unit Delay1/1 -> MATLAB Function/2(I)
  MATLAB Function/1(Vref) -> Sum8/1
  Bus Selector/2 -> [Ipv]  "<I_PV>"
  Demux5/3 -> Relay/3(In3)
  Demux5/1 -> Relay/1(In1)
  Relay/1(Out1) -> Three-Phase Breaker/1
  Demux5/2 -> Relay/2(In2)
  Unit Delay2/1 -> Demux5/1
  RMS/1 -> Display/1
  Three-Phase V-I Measurement2/2 -> RMS/1, Unit Delay2/1, Scope/2
  Demux4/1 -> Scope13/1
  Demux4/2 -> Scope13/2
  Demux6/3 -> Scope14/3
  Demux6/2 -> Scope14/2
  Demux6/1 -> Scope14/1
  abc to Alpha-Beta-Zero/1 -> Alpha-Beta-Zero to dq0/1, Demux6/1, Scope1/3, [alphabeta]
  Demux4/3 -> Scope13/3
  [Solar_Vabc] -> abc to Alpha-Beta-Zero/1, Scope1/4, Demux7/1
  Demux7/1 -> Scope15/1
  Demux7/2 -> Scope15/2
  Demux7/3 -> Scope15/3
  Alpha-Beta-Zero to dq1/1 -> Demux8/1, Scope8/2, Demux2/1
  Demux8/1 -> Scope16/1
  Demux8/2 -> Scope16/2
  Demux8/3 -> Scope16/3
  Demux9/3 -> Scope17/3
  Demux9/2 -> Scope17/2
  Demux9/1 -> Scope17/1
  Demux10/3 -> Scope18/3
  Demux10/2 -> Scope18/2
  Demux10/1 -> Scope18/1
  Demux11/1 -> Scope19/1
  Demux11/2 -> Scope19/2
  Demux11/3 -> Scope19/3
  abc to dq0/1 -> Demux11/1, Scope7/3, Demux1/1
  Constant/1 -> PV Array/1
  Constant1/1 -> PV Array/2
  connections:
  Series RLC Branch7/LConn1 -- Series RLC Branch4/LConn1 -- Series RLC Branch1/RConn1
  Three-Phase V-I Measurement2/LConn1 -- Three-Phase Transformer (Two Windings)/RConn1 -- Three-Phase Series RLC Load/LConn1
  Series RLC Branch6/LConn1 -- Series RLC Branch3/LConn1 -- Series RLC Branch/RConn1
  Three-Phase V-I Measurement1/LConn3 -- Three-Phase Transformer (Two Windings)/LConn3
  Series RLC Branch7/RConn1 -- Series RLC Branch8/RConn1 -- Series RLC Branch6/RConn1
  Series RLC Branch/LConn1 -- Three-Phase V-I Measurement/RConn1
  Series RLC Branch8/LConn1 -- Series RLC Branch5/LConn1 -- Series RLC Branch2/RConn1
  Series RLC Branch3/RConn1 -- Three-Phase V-I Measurement1/RConn1
  Three-Phase V-I Measurement2/LConn2 -- Three-Phase Transformer (Two Windings)/RConn2 -- Three-Phase Series RLC Load/LConn2
  Three-Phase V-I Measurement2/LConn3 -- Three-Phase Transformer (Two Windings)/RConn3 -- Three-Phase Series RLC Load/LConn3
  Series RLC Branch9/LConn1 -- PV Array/RConn1 -- Series RLC Branch10/RConn1
  Series RLC Branch5/RConn1 -- Three-Phase V-I Measurement1/RConn3
  Three-Phase V-I Measurement1/LConn1 -- Three-Phase Transformer (Two Windings)/LConn1
  Series RLC Branch2/LConn1 -- Three-Phase V-I Measurement/RConn3
  Series RLC Branch4/RConn1 -- Three-Phase V-I Measurement1/RConn2
  IGBT/Diode3/RConn1 -- PV Array/RConn2 -- Series RLC Branch9/RConn1 -- IGBT/Diode6/RConn1 -- Series RLC Branch11/LConn1 -- Voltage Measurement/LConn2 -- IGBT/Diode5/RConn1 -- IGBT/Diode4/RConn1
  Three-Phase V-I Measurement1/LConn2 -- Three-Phase Transformer (Two Windings)/LConn2
  Series RLC Branch1/LConn1 -- Three-Phase V-I Measurement/RConn2
  IGBT/Diode3/LConn1 -- Three-Phase V-I Measurement/LConn1 -- IGBT/Diode/RConn1
  IGBT/Diode4/LConn1 -- IGBT/Diode1/RConn1 -- Three-Phase V-I Measurement/LConn2
  IGBT/Diode5/LConn1 -- IGBT/Diode2/RConn1 -- Three-Phase V-I Measurement/LConn3
  Diode/LConn1 -- Series RLC Branch10/LConn1 -- IGBT/Diode6/LConn1
  IGBT/Diode/LConn1 -- IGBT/Diode2/LConn1 -- IGBT/Diode1/LConn1 -- Voltage Measurement/LConn1 -- Series RLC Branch11/RConn1 -- Diode/RConn1
  Connection Port/RConn1 -- Three-Phase Breaker/LConn1
  Three-Phase Breaker/LConn2 -- Connection Port1/RConn1
  Three-Phase Breaker/LConn3 -- Connection Port2/RConn1
  Three-Phase Breaker/RConn1 -- Three-Phase V-I Measurement2/RConn1
  Three-Phase V-I Measurement2/RConn2 -- Three-Phase Breaker/RConn2
  Three-Phase V-I Measurement2/RConn3 -- Three-Phase Breaker/RConn3

== system Smart_Grid_2/Wind_Farm 48KW ==
  Wind_Turbine 1 : Subsystem
      mask Display: image('Horizontal axis wind turbine.jpg');
  Wind_Turbine 2 : Subsystem
      mask Display: image('Horizontal axis wind turbine.jpg');
  Wind_Turbine 3 : Subsystem
      mask Display: image('Horizontal axis wind turbine.jpg');
  Wind_Turbine 4 : Subsystem
      mask Display: image('Horizontal axis wind turbine.jpg');
  Connection Port : PMIOPort  Side=Right
  Connection Port1 : PMIOPort  Port=2  Side=Right
  Connection Port2 : PMIOPort  Port=3  Side=Right
  connections:
  Wind_Turbine 4/RConn1 -- Wind_Turbine 3/RConn1 -- Connection Port/RConn1 -- Wind_Turbine 1/RConn1 -- Wind_Turbine 2/RConn1
  Wind_Turbine 4/RConn2 -- Wind_Turbine 3/RConn2 -- Connection Port1/RConn1 -- Wind_Turbine 1/RConn2 -- Wind_Turbine 2/RConn2
  Wind_Turbine 4/RConn3 -- Wind_Turbine 3/RConn3 -- Connection Port2/RConn1 -- Wind_Turbine 1/RConn3 -- Wind_Turbine 2/RConn3

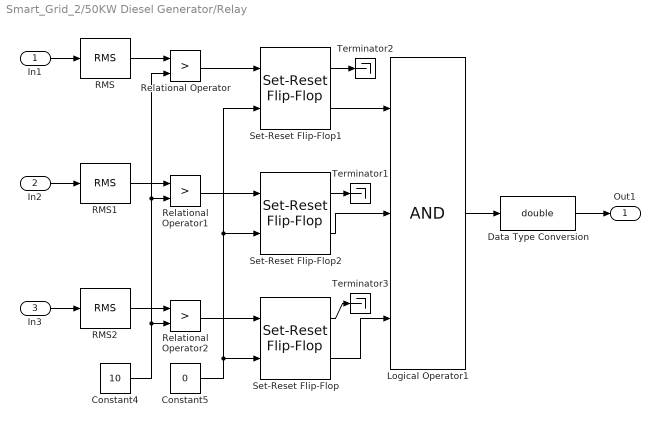
== system Smart_Grid_2/50KW Diesel Generator/Relay ==
  In1 : Inport
  In2 : Inport  Port=2
  In3 : Inport  Port=3
  Constant4 : Constant  Value=10
  Constant5 : Constant  Value=0
  Data Type Conversion : DataTypeConversion  OutDataTypeStr=double  SaturateOnIntegerOverflow=off  RndMeth=Floor
  Logical Operator1 : Logic  Inputs=3  AllPortsSameDT=off  OutDataTypeStr=boolean
  RMS : spsRMSLib/RMS  TrueRMS=on  Freq=50  RMSInit=0  Ts=0.001
  RMS1 : spsRMSLib/RMS  TrueRMS=on  Freq=50  RMSInit=0  Ts=0.001
  RMS2 : spsRMSLib/RMS  TrueRMS=on  Freq=50  RMSInit=0  Ts=0.001
  Relational Operator : RelationalOperator  Operator=>  OutDataTypeStr=boolean  RndMeth=Simplest  InputSameDT=off
  Relational Operator1 : RelationalOperator  Operator=>  OutDataTypeStr=boolean  RndMeth=Simplest  InputSameDT=off
  Relational Operator2 : RelationalOperator  Operator=>  OutDataTypeStr=boolean  RndMeth=Simplest  InputSameDT=off
  Set-Reset Flip-Flop : eeGeneralControl/Set-Reset Flip-Flop  LabelModeActiveChoice=Discrete  UndefState=Set  Q0=0  Ts=0.001
  Set-Reset Flip-Flop1 : eeGeneralControl/Set-Reset Flip-Flop  LabelModeActiveChoice=Discrete  UndefState=Set  Q0=0  Ts=0.001
  Set-Reset Flip-Flop2 : eeGeneralControl/Set-Reset Flip-Flop  LabelModeActiveChoice=Discrete  UndefState=Reset  Q0=0  Ts=0.001
  Terminator1 : Terminator
  Terminator2 : Terminator
  Terminator3 : Terminator
  Out1 : Outport
  wires:
  In2/1 -> RMS1/1
  Relational Operator1/1 -> Set-Reset Flip-Flop2/1
  Constant4/1 -> Relational Operator/2, Relational Operator1/2, Relational Operator2/2
  Constant5/1 -> Set-Reset Flip-Flop1/2, Set-Reset Flip-Flop2/2, Set-Reset Flip-Flop/2
  Logical Operator1/1 -> Data Type Conversion/1
  Data Type Conversion/1 -> Out1/1
  In3/1 -> RMS2/1
  In1/1 -> RMS/1
  RMS1/1 -> Relational Operator1/1
  RMS2/1 -> Relational Operator2/1
  RMS/1 -> Relational Operator/1
  Relational Operator2/1 -> Set-Reset Flip-Flop/1
  Relational Operator/1 -> Set-Reset Flip-Flop1/1
  Set-Reset Flip-Flop/2 -> Logical Operator1/3
  Set-Reset Flip-Flop2/2 -> Logical Operator1/2
  Set-Reset Flip-Flop1/2 -> Logical Operator1/1
  Set-Reset Flip-Flop2/1 -> Terminator1/1
  Set-Reset Flip-Flop/1 -> Terminator3/1
  Set-Reset Flip-Flop1/1 -> Terminator2/1

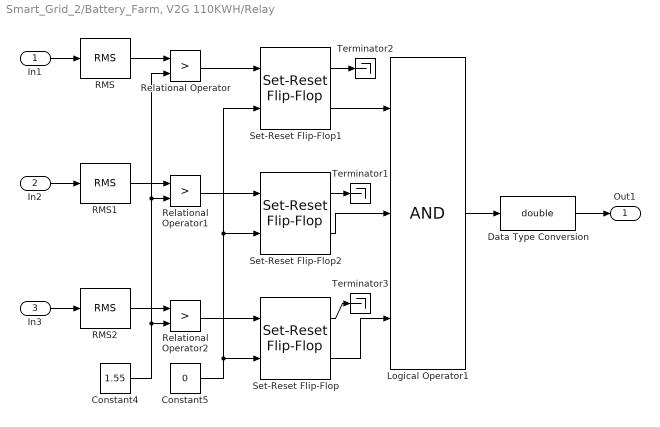
== system Smart_Grid_2/Battery_Farm, V2G 110KWH/Relay ==
  In1 : Inport
  In2 : Inport  Port=2
  In3 : Inport  Port=3
  Constant4 : Constant  Value=1.55
  Constant5 : Constant  Value=0
  Data Type Conversion : DataTypeConversion  OutDataTypeStr=double  SaturateOnIntegerOverflow=off  RndMeth=Floor
  Logical Operator1 : Logic  Inputs=3  AllPortsSameDT=off  OutDataTypeStr=boolean
  RMS : spsRMSLib/RMS  TrueRMS=on  Freq=50  RMSInit=0  Ts=0.001
  RMS1 : spsRMSLib/RMS  TrueRMS=on  Freq=50  RMSInit=0  Ts=0.001
  RMS2 : spsRMSLib/RMS  TrueRMS=on  Freq=50  RMSInit=0  Ts=0.001
  Relational Operator : RelationalOperator  Operator=>  OutDataTypeStr=boolean  RndMeth=Simplest  InputSameDT=off
  Relational Operator1 : RelationalOperator  Operator=>  OutDataTypeStr=boolean  RndMeth=Simplest  InputSameDT=off
  Relational Operator2 : RelationalOperator  Operator=>  OutDataTypeStr=boolean  RndMeth=Simplest  InputSameDT=off
  Set-Reset Flip-Flop : eeGeneralControl/Set-Reset Flip-Flop  LabelModeActiveChoice=Discrete  UndefState=Set  Q0=0  Ts=0.001
  Set-Reset Flip-Flop1 : eeGeneralControl/Set-Reset Flip-Flop  LabelModeActiveChoice=Discrete  UndefState=Set  Q0=0  Ts=0.001
  Set-Reset Flip-Flop2 : eeGeneralControl/Set-Reset Flip-Flop  LabelModeActiveChoice=Discrete  UndefState=Reset  Q0=0  Ts=0.001
  Terminator1 : Terminator
  Terminator2 : Terminator
  Terminator3 : Terminator
  Out1 : Outport
  wires:
  In2/1 -> RMS1/1
  Relational Operator1/1 -> Set-Reset Flip-Flop2/1
  Constant4/1 -> Relational Operator/2, Relational Operator1/2, Relational Operator2/2
  Constant5/1 -> Set-Reset Flip-Flop1/2, Set-Reset Flip-Flop2/2, Set-Reset Flip-Flop/2
  Logical Operator1/1 -> Data Type Conversion/1
  Data Type Conversion/1 -> Out1/1
  In3/1 -> RMS2/1
  In1/1 -> RMS/1
  RMS1/1 -> Relational Operator1/1
  RMS2/1 -> Relational Operator2/1
  RMS/1 -> Relational Operator/1
  Relational Operator2/1 -> Set-Reset Flip-Flop/1
  Relational Operator/1 -> Set-Reset Flip-Flop1/1
  Set-Reset Flip-Flop/2 -> Logical Operator1/3
  Set-Reset Flip-Flop2/2 -> Logical Operator1/2
  Set-Reset Flip-Flop1/2 -> Logical Operator1/1
  Set-Reset Flip-Flop2/1 -> Terminator1/1
  Set-Reset Flip-Flop/1 -> Terminator3/1
  Set-Reset Flip-Flop1/1 -> Terminator2/1
